simulink model "flattening_4_test"  (Simulink 7.2)
settings: Solver=ode45  StartTime=0.0  StopTime=10.0  RelTol=1e-3
settings Model: Creator=arnaud  LastModifiedBy=arnaud

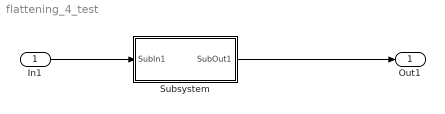
== system flattening_4_test ==
  In1 : Inport  OutDataType=sfix(16)  OutScaling=2^0
  Subsystem : Subsystem
  Out1 : Outport  OutDataType=sfix(16)  OutScaling=2^0
  wires:
  In1/1 -> Subsystem/1(SubIn1)
  Subsystem/1(SubOut1) -> Out1/1

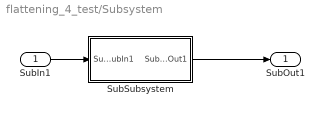
== system flattening_4_test/Subsystem ==
  SubIn1 : Inport  OutDataType=sfix(16)  OutScaling=2^0
  SubSubsystem : Subsystem
  SubOut1 : Outport  OutDataType=sfix(16)  OutScaling=2^0
  wires:
  SubIn1/1 -> SubSubsystem/1(SubSubIn1)
  SubSubsystem/1(SubSubOut1) -> SubOut1/1

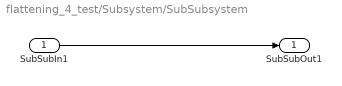
== system flattening_4_test/Subsystem/SubSubsystem ==
  SubSubIn1 : Inport  OutDataType=sfix(16)  OutScaling=2^0
  SubSubOut1 : Outport  OutDataType=sfix(16)  OutScaling=2^0
  wires:
  SubSubIn1/1 -> SubSubOut1/1
